simulink model "bumpless_control"  (Simulink 3.00)
libraries: mathlib x10, reglib x3, execlib x2, analoglib x1, arclib x1

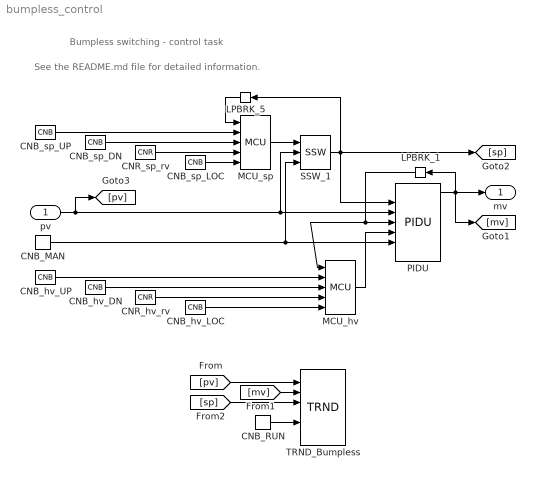
== system bumpless_control ==
  note: See the README.md file for detailed information.
  note: Bumpless switching - control task
  pv : Inport  Port=1
  CNB_MAN : mathlib/CNB  YCN=off
  CNB_RUN : mathlib/CNB  YCN=on
  CNB_hv_DN : mathlib/CNB  YCN=off
  CNB_hv_LOC : mathlib/CNB  YCN=on
  CNB_hv_UP : mathlib/CNB  YCN=off
  CNB_sp_DN : mathlib/CNB  YCN=off
  CNB_sp_LOC : mathlib/CNB  YCN=on
  CNB_sp_UP : mathlib/CNB  YCN=off
  CNR_hv_rv : mathlib/CNR  ycn=0
  CNR_sp_rv : mathlib/CNR  ycn=0
  LPBRK_1 : execlib/LPBRK  Orientation=left
  LPBRK_5 : execlib/LPBRK  Orientation=left
  MCU_hv : reglib/MCU  tt=1  tm=100  y0=0  q=5  ta=4  tf=8  SATF=on  hilim=1  lolim=-1
  MCU_sp : reglib/MCU  tt=1  tm=100  y0=0  q=5  ta=4  tf=8  SATF=on  hilim=1  lolim=-1
  PIDU : reglib/PIDU  irtype=7: PID  RACT=off  k=0.6  ti=4  td=1  nd=10  b=1  c=0  tt=1  hilim=1  lolim=-1  dz=0  icotype=1: Analog
  SSW_1 : analoglib/SSW
  TRND_Bumpless : arclib/TRND  n=3  l=1000  btype=8: Double  ptype1=1: Store  ptype2=1: Store  ptype3=1: Store  ptype4=1: Store  pfac=1  afac=0  arc=0  id=1  Title=Trend Title  timesrc=1
  mv : Outport  Port=1
  wires:
  CNB_MAN/1 -> PIDU/6, SSW_1/3
  CNB_RUN/1 -> TRND_Bumpless/5
  CNB_hv_DN/1 -> MCU_hv/3
  CNB_hv_LOC/1 -> MCU_hv/5
  CNB_hv_UP/1 -> MCU_hv/2
  CNB_sp_DN/1 -> MCU_sp/3
  CNB_sp_LOC/1 -> MCU_sp/5
  CNB_sp_UP/1 -> MCU_sp/2
  CNR_hv_rv/1 -> MCU_hv/4
  CNR_sp_rv/1 -> MCU_sp/4
  [pv] -> TRND_Bumpless/1
  [mv] -> TRND_Bumpless/2
  [sp] -> TRND_Bumpless/3
  LPBRK_1/1 -> MCU_hv/1, PIDU/4
  LPBRK_5/1 -> MCU_sp/1
  MCU_hv/1 -> PIDU/5
  MCU_sp/1 -> SSW_1/1
  PIDU/1 -> [mv], LPBRK_1/1, mv/1
  SSW_1/1 -> [sp], LPBRK_5/1, PIDU/2
  pv/1 -> PIDU/3, SSW_1/2, [pv]
